simulink model "lab_7_simulink"  (R2021b)
settings: Solver=VariableStepAuto  StartTime=0.0  StopTime=20  RelTol=1e-3
settings Model: Creator=rcmas  LastModifiedBy=rcmas

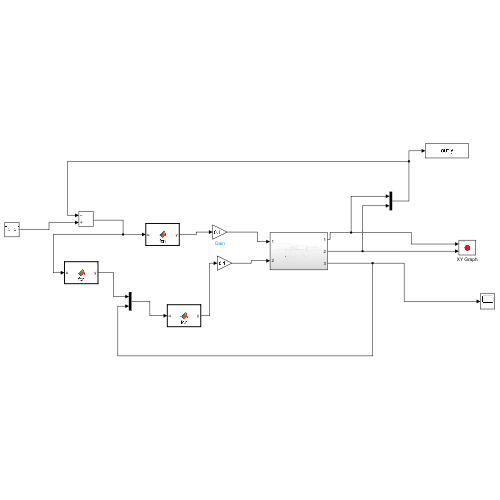
[thumbnail: Simulink's stored preview of the top-level diagram]
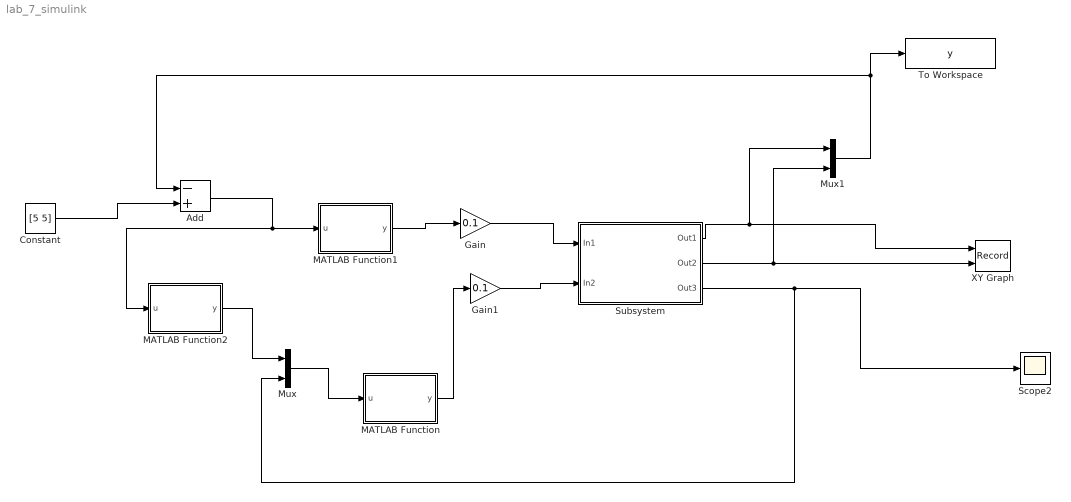
== system lab_7_simulink ==
  Add : Sum  Inputs=-+
  Constant : Constant  Value=[5 5]
  Gain : Gain  Gain=0.1
  Gain1 : Gain  Gain=0.1
  MATLAB Function : MATLAB Function  TreatAsAtomicUnit=on
  MATLAB Function1 : MATLAB Function  Tag=sqrt  TreatAsAtomicUnit=on
  MATLAB Function2 : MATLAB Function  TreatAsAtomicUnit=on
  Mux : Mux  Inputs=2
  Mux1 : Mux  Inputs=2
  Scope2 : Scope
  Subsystem : Subsystem
  To Workspace : ToWorkspace  VariableName=y  SaveFormat=Timeseries  SampleTime=-1
  XY Graph : Record  FileSettingsInternal="{\"entries\":[{\"content\":{\"excelSettings\":{\"content\":{},\"type\":\"Streamout.ExcelSettings\"}},\"type\":\"Streamout.FileSettingStorage\",\"uuid\":\"2433149c-eb71-4d90-91f5-c6a0c2d4525a\"}],\"packageUris\":[\"http://schema.mathworks.com/mf0/streamout_blocks/R2020a\"],\"version\":\"1.0\"}"  Layout=[1 1]  SignalsInternal="{\"entries\":[{\"content\":{\"signals\":[{\"content\":{\"blockPath\":[\"lab_7_simulink/XY Graph\"],\"channel\":[],\"dimensions\":[1],\"domain\":\"lab_7_simulink/XY Graph\",\"lineColor\":\"#a2142f\",\"plots\":[1],\"port\":1,\"sid\":[\"\"],\"signalID\":264,\"signalName\":\"Subsystem:1\"},\"type\":\"RecordBlkView.Signal\",\"uuid\":\"97195364-4181-4a20-9340-e71fbb45bf0b\"},{\"content\":{\"blockPath\":[\"lab_7_simulink/XY Graph\"],\"channel\":[],\"dimensions\":[1],\"domain\":\"lab_7_simulink/XY Graph\",\"lineColor\":\"#139fff\",\"plots\":[1],\"port\":2,\"sid\":[\"\"],\"signalID\":268,\"signalName\":\"Subsystem:2\"},\"type\":\"RecordBlkView.Signal\",\"uuid\":\"f91adedf-864c-416c-82fb-acd01aed0b8b\"}]},\"type\":\"RecordBlkView.InputSignals\",\"uuid\":\"787416bb-d7f2-44b3-b3f0-71e17baef33b\"}],\"packageUris\":[\"http://schema.mathworks.com/mf0/streamout_blocks/R2020a\"],\"version\":\"1.0\"}"  VisualizationBindings="{\"xyplotplugin\":{\"info\":[{\"series\":[{\"bindingParametersList\":[{\"parameter\":\"X-Axis\",\"signalID\":264,\"signalName\":\"Subsystem:1\"},{\"parameter\":\"Y-Axis\",\"signalID\":268,\"signalName\":\"Subsystem:2\"}],\"seriesID\":36280}],\"subplotID\":1}]}}"  CompatibilityTag=XY
  wires:
  Subsystem/1(Out1) -> Mux1/1, XY Graph/1
  Subsystem/2(Out2) -> Mux1/2, XY Graph/2
  Subsystem/3(Out3) -> Mux/2, Scope2/1
  Mux/1 -> MATLAB Function/1(u)
  MATLAB Function2/1(y) -> Mux/1
  Add/1 -> MATLAB Function1/1(u), MATLAB Function2/1(u)
  MATLAB Function1/1(y) -> Gain/1
  Gain/1 -> Subsystem/1(In1)
  Gain1/1 -> Subsystem/2(In2)
  MATLAB Function/1(y) -> Gain1/1
  Constant/1 -> Add/2
  Mux1/1 -> Add/1, To Workspace/1

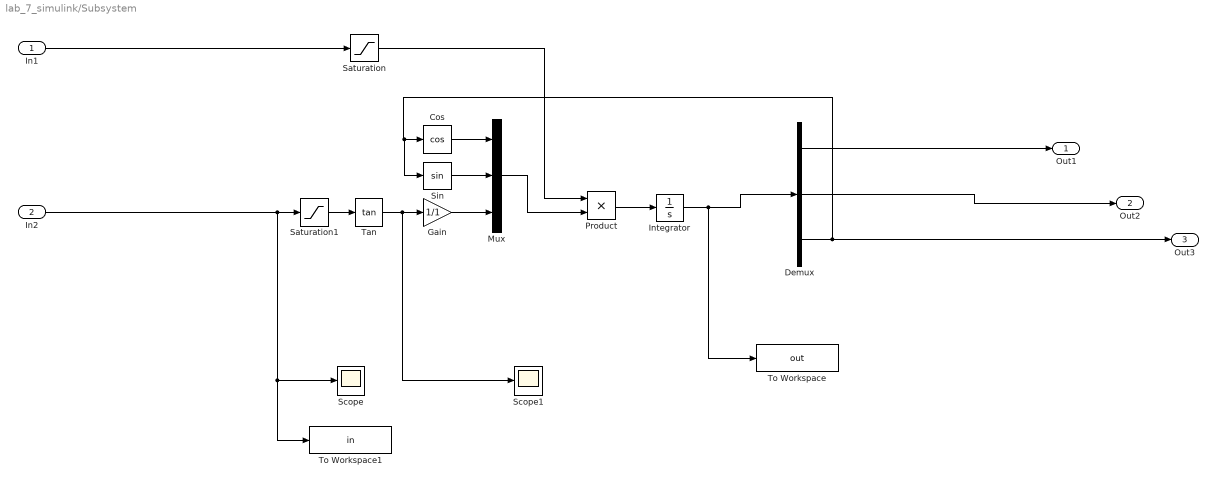
== system lab_7_simulink/Subsystem ==
  In1 : Inport
  In2 : Inport  Port=2
  Cos : Trigonometry  Operator=cos
  Demux : Demux  Outputs=3
  Gain : Gain  Gain=1/1
  Integrator : Integrator  InitialCondition=[8 5 pi/2]
  Mux : Mux  Inputs=3
  Product : Product
  Saturation : Saturate
  Saturation1 : Saturate
  Scope : Scope
  Scope1 : Scope
  Sin : Trigonometry
  Tan : Trigonometry  Operator=tan
  To Workspace : ToWorkspace  VariableName=out  SaveFormat=Timeseries  SampleTime=-1
  To Workspace1 : ToWorkspace  VariableName=in  SaveFormat=Timeseries  SampleTime=-1
  Out1 : Outport
  Out2 : Outport  Port=2
  Out3 : Outport  Port=3
  wires:
  Demux/1 -> Out1/1
  In1/1 -> Saturation/1
  Gain/1 -> Mux/3
  In2/1 -> To Workspace1/1, Scope/1, Saturation1/1
  Tan/1 -> Scope1/1, Gain/1
  Sin/1 -> Mux/2
  Saturation/1 -> Product/1
  Saturation1/1 -> Tan/1
  Mux/1 -> Product/2
  Integrator/1 -> To Workspace/1, Demux/1
  Demux/2 -> Out2/1
  Demux/3 -> Out3/1, Sin/1, Cos/1
  Product/1 -> Integrator/1
  Cos/1 -> Mux/1

== matlab function lab_7_simulink/MATLAB Function ==
  data: u input; y output
function y = fcn(u)

y = angdiff(u(2), u(1));

== matlab function lab_7_simulink/MATLAB Function2 ==
  data: u input; y output
function y = fcn(u)

y = atan2(u(2), u(1));

== matlab function lab_7_simulink/MATLAB Function1 ==
  data: u input; y output
function y = fcn(u)

y = sqrt(u(1)^2 + u(2)^2);
